simulink model "simulation_ex6"  (R2023a)
settings: Solver=VariableStepAuto  StartTime=0.0  StopTime=10  RelTol=1e-3
settings Model: Creator=vigro  LastModifiedBy=vigro
settings DataIOCC: ReturnWorkspaceOutputs=off

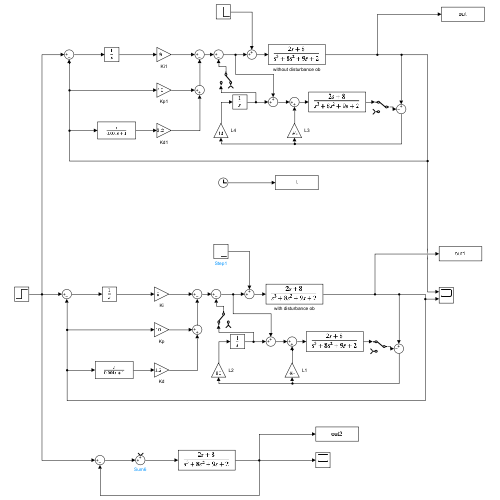
[thumbnail: Simulink's stored preview of the top-level diagram]
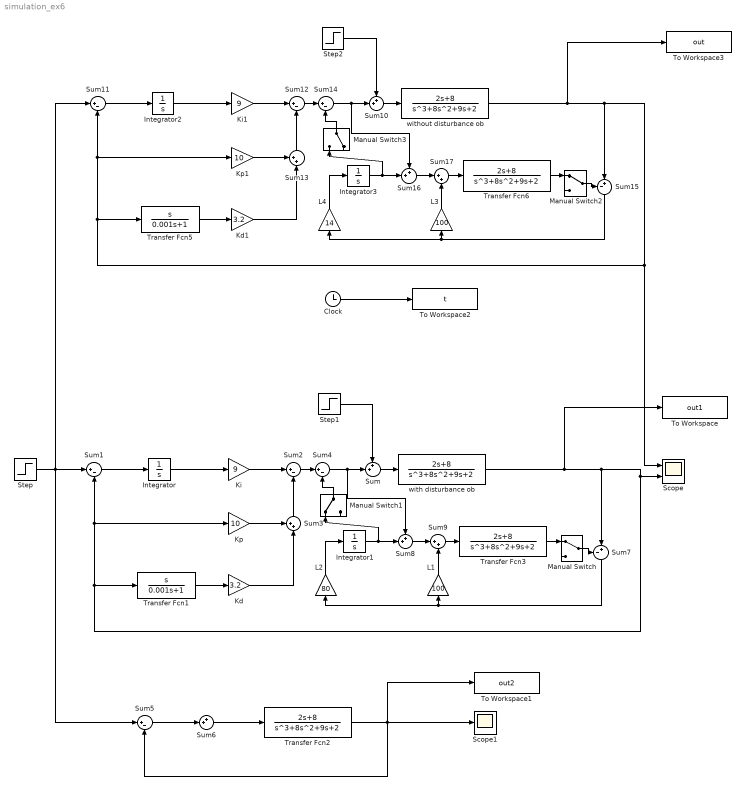
== system simulation_ex6 ==
  Clock : Clock
  Integrator{,1..3} (4 alike) : Integrator
  Kd : Gain  Gain=3.2
  Kd1 : Gain  Gain=3.2
  Ki : Gain  Gain=9
  Ki1 : Gain  Gain=9
  Kp : Gain  Gain=10
  Kp1 : Gain  Gain=10
  L1 : Gain  Gain=100
  L2 : Gain  Gain=80
  L3 : Gain  Gain=100
  L4 : Gain  Gain=14
  Manual Switch : ManualSwitch
  Manual Switch1 : ManualSwitch
  Manual Switch2 : ManualSwitch
  Manual Switch3 : ManualSwitch  CurrentSetting=0
  Scope : Scope  NumInputPorts=2
  Scope1 : Scope
  Step : Step  Time=2  SampleTime=0
  Step1 : Step  Time=6  After=-2  SampleTime=0
  Step2 : Step  Time=6  After=-2  SampleTime=0
  Sum{,3,6,8,10,13,16} (7 alike) : Sum  Inputs=++|
  Sum{1..2,4..5,11..12,14} (7 alike) : Sum  Inputs=|+-
  Sum15 : Sum  Inputs=-+|
  Sum17 : Sum  Inputs=|++
  Sum7 : Sum  Inputs=-+|
  Sum9 : Sum  Inputs=|++
  To Workspace : ToWorkspace  VariableName=out1  SaveFormat=Timeseries  SampleTime=-1
  To Workspace1 : ToWorkspace  VariableName=out2  SaveFormat=Timeseries  SampleTime=-1
  To Workspace2 : ToWorkspace  VariableName=t  SaveFormat=Timeseries  SampleTime=-1
  To Workspace3 : ToWorkspace  VariableName=out  SaveFormat=Timeseries  SampleTime=-1
  Transfer Fcn1 : TransferFcn  Numerator=[1 0]  Denominator=[0.001 1]
  Transfer Fcn2 : TransferFcn  Numerator=[2 8]  Denominator=[1 8 9 2]
  Transfer Fcn3 : TransferFcn  Numerator=[2 8]  Denominator=[1 8 9 2]
  Transfer Fcn5 : TransferFcn  Numerator=[1 0]  Denominator=[0.001 1]
  Transfer Fcn6 : TransferFcn  Numerator=[2 8]  Denominator=[1 8 9 2]
  with disturbance ob : TransferFcn  Numerator=[2 8]  Denominator=[1 8 9 2]
  without disturbance ob : TransferFcn  Numerator=[2 8]  Denominator=[1 8 9 2]
  wires:
  Step/1 -> Sum11/1, Sum5/1, Sum1/1
  Sum1/1 -> Integrator/1
  Integrator/1 -> Ki/1
  Ki/1 -> Sum2/1
  Sum/1 -> with disturbance ob/1
  Kp/1 -> Sum3/1
  Sum3/1 -> Sum2/2
  Kd/1 -> Sum3/2
  Transfer Fcn1/1 -> Kd/1
  with disturbance ob/1 -> Sum7/2, Transfer Fcn1/1, Kp/1, Sum1/2, Scope/2, To Workspace/1
  Sum2/1 -> Sum4/1
  Sum4/1 -> Sum8/1, Sum/2
  Transfer Fcn2/1 -> Scope1/1, To Workspace1/1, Sum5/2
  Clock/1 -> To Workspace2/1
  Step1/1 -> Sum/1
  Sum5/1 -> Sum6/2
  Sum6/1 -> Transfer Fcn2/1
  Transfer Fcn3/1 -> Manual Switch/1
  Manual Switch/1 -> Sum7/1
  Integrator1/1 -> Manual Switch1/1, Sum8/2
  L2/1 -> Integrator1/1
  Sum7/1 -> L2/1, L1/1
  Manual Switch1/1 -> Sum4/2
  Sum9/1 -> Transfer Fcn3/1
  Sum8/1 -> Sum9/1
  L1/1 -> Sum9/2
  Sum16/1 -> Sum17/1
  L3/1 -> Sum17/2
  Sum15/1 -> L4/1, L3/1
  Step2/1 -> Sum10/1
  Manual Switch3/1 -> Sum14/2
  Manual Switch2/1 -> Sum15/1
  Transfer Fcn6/1 -> Manual Switch2/1
  L4/1 -> Integrator3/1
  Sum12/1 -> Sum14/1
  without disturbance ob/1 -> Sum15/2, Scope/1, Transfer Fcn5/1, Kp1/1, Sum11/2, To Workspace3/1
  Sum10/1 -> without disturbance ob/1
  Sum17/1 -> Transfer Fcn6/1
  Sum13/1 -> Sum12/2
  Integrator2/1 -> Ki1/1
  Kp1/1 -> Sum13/1
  Sum11/1 -> Integrator2/1
  Integrator3/1 -> Manual Switch3/1, Sum16/2
  Transfer Fcn5/1 -> Kd1/1
  Kd1/1 -> Sum13/2
  Sum14/1 -> Sum16/1, Sum10/2
  Ki1/1 -> Sum12/1
